simulink model "Copy_of_modele"  (R2025b)
settings: Solver=VariableStepAuto  StartTime=0.0  StopTime=100  RelTol=1e-3
values from neighbouring files (symbols this model uses):
  Axy = 0.0    (= 0)    [PropKtKq.m]    (also in variables_procom.m = prop.Axy)
  Cxy = 0.0    (= 0)    [PropKtKq.m]    (also in variables_procom.m = prop.Cxy)
  D = 0.0    (= 0)    [PropKtKq.m]    (also in variables_procom.m = prop.D)
  eta_mt = 0.4    [variables_procom.m]
  Jprop = Jmt/R^2    (= 19.35886398)    [variables_procom.m]
  m = 0.0    (= 0)    [Hulldyn.m]    (also in variables_procom.m = 250000)
  ma = 123434    [variables_procom.m]
  Pe = 5    [variables_procom.m]
  Py = 60    [variables_procom.m]
  R = 1/2.953    (= 0.338638672536)    [variables_procom.m]
  tau_mt = 0.4    [variables_procom.m]
  Tc = 0.0    (= 0)    [Hulldyn.m]    (also in variables_procom.m = 5800)
  th = 0.0    (= 0)    [Hulldyn.m]    (also in PropKtKq.m; variables_procom.m = hull.th)
  wh = 0.0    (= 0)    [Hulldyn.m]    (also in PropKtKq.m; variables_procom.m = hull.wh)
  x = 0.0    (= 0)    [PropKtKq.m]    (also in variables_procom.m = prop.x)
  y = 0.0    (= 0)    [PropKtKq.m]    (also in variables_procom.m = prop.y)
libraries: slpidlib x1
settings Model: Creator=leagr  LastModifiedBy=flo

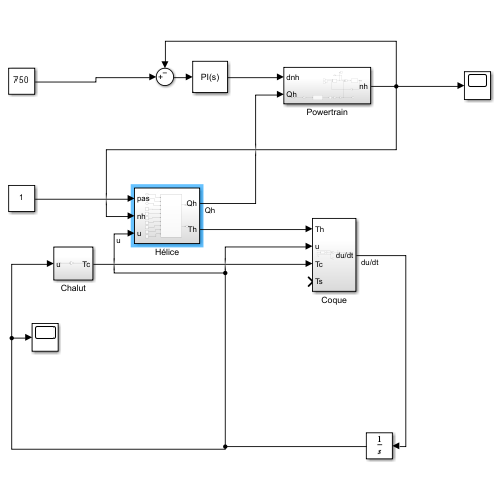
[thumbnail: Simulink's stored preview of the top-level diagram]
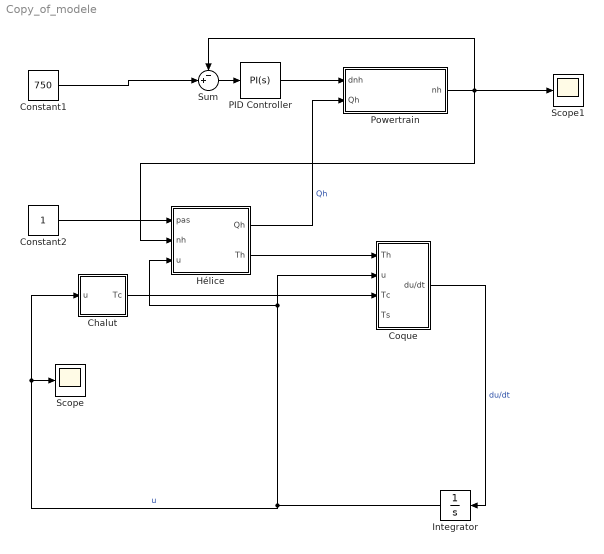
== system Copy_of_modele ==
  Chalut : Subsystem
  Constant1 : Constant  Value=750
  Constant2 : Constant
  Coque : Subsystem
  Hélice : Subsystem
  Integrator : Integrator
  PID Controller : slpidlib/PID Controller  Controller=PI  Form=Parallel  TimeDomain=Continuous-time  UseExternalTs=off  SampleTime=-1  IntegratorMethod=Forward Euler  FilterMethod=Forward Euler  ControllerParametersSource=internal  P=2.47620344962392  I=0.00577839793928918  UseKiTs=off  D=0  UseExternalDerivativeSource=off  N=100  UseFilter=on  TunerSelectOption=Transfer Function Based (PID Tuner App)  InitialConditionSource=internal  InitialConditionForIntegrator=0  InitialConditionForFilter=0  DifferentiatorICPrevScaledInput=0  ExternalReset=none  TrackingMode=off  Kt=1  LimitOutput=off  SatLimitsSource=internal  UpperSaturationLimit=inf  LowerSaturationLimit=-inf  LinearizeAsGain=on  AntiWindupMode=none  Kb=1  LimitIntegrator=off  UpperIntegratorSaturationLimit=inf  LowerIntegratorSaturationLimit=-inf  POutMin=[]  POutMax=[]  IOutMin=[]  IOutMax=[]  DOutMin=[]  DOutMax=[]  NOutMin=[]  NOutMax=[]  SumOutMin=[]  SumOutMax=[]  SaturationOutMin=[]  SaturationOutMax=[]  PParamMin=[]  PParamMax=[]  IParamMin=[]  IParamMax=[]  DParamMin=[]  DParamMax=[]  NParamMin=[]  NParamMax=[]  KbParamMin=[]  KbParamMax=[]  KtParamMin=[]  KtParamMax=[]  KbOutMin=[]  KbOutMax=[]  KtOutMin=[]  KtOutMax=[]  IntegratorOutMin=[]  IntegratorOutMax=[]  FilterOutMin=[]  FilterOutMax=[]  SumI1OutMin=[]  SumI1OutMax=[]  SumI2OutMin=[]  SumI2OutMax=[]  SumI3OutMin=[]  SumI3OutMax=[]  SumI4OutMin=[]  SumI4OutMax=[]  SumDOutMin=[]  SumDOutMax=[]  DifferentiatorOutMin=[]  DifferentiatorOutMax=[]  FilterDiffOutCoefMin=[]  FilterDiffOutCoefMax=[]  ReciprocalOutMin=[]  ReciprocalOutMax=[]  SumDenOutMin=[]  SumDenOutMax=[]  SumNumOutMin=[]  SumNumOutMax=[]  DivideOutMin=[]  DivideOutMax=[]  UdiffTsProdOutMin=[]  UdiffTsProdOutMax=[]  NTsProdOutMin=[]  NTsProdOutMax=[]  UintegralTsProdOutMin=[]  UintegralTsProdOutMax=[]  UngainTsProdOutMin=[]  UngainTsProdOutMax=[]  ClampingZeroOutDataTypeStr=Inherit: Inherit via back propagation  ClampingZeroOutMin=[]  ClampingZeroOutMax=[]  FilterDenConstantOutDataTypeStr=Inherit: Inherit via back propagation  FilterDenConstantOutMin=[]  FilterDenConstantOutMax=[]  PCopyOutDataTypeStr=Inherit: Inherit via back propagation  PCopyOutMin=[]  PCopyOutMax=[]  NCopyOutDataTypeStr=Inherit: Inherit via back propagation  NCopyOutMin=[]  NCopyOutMax=[]  IntegratorContinuousStateAttributes=''  IntegratorStateMustResolveToSignalObject=off  IntegratorRTWStateStorageClass=Auto  FilterContinuousStateAttributes=''  FilterStateMustResolveToSignalObject=off  FilterRTWStateStorageClass=Auto  ParallelPVariant=InternalParameters  IdealPVariant=Disabled  IVariant=InternalParameters  DVariant=Disabled  IntegratorVariant=Continuous  SatVariant=Disabled  AWVariant=Passthrough  PCopyVariant=Disabled  TRVariant=Disabled  FdbkBlocksVariant=Forward  IdealPFdbkVariant=Disabled  SatFdbkVariant=Disabled  DerivativeFilterVariant=Disabled  NVariant=Disabled  NCopyVariant=Disabled_SignalSpec  FilterICVariant=Disabled  IntegratorICVariant=InternalICs  ExternalResetVariant=Disabled  TRSumVariant=Passthrough  SumFdbkVariant=Disabled  SumVariant=Sum_PI  TsampFilterVariant=InternalTs  TsampNgainVariant=Passthrough  TsampIntegralVariant=Disabled_SignalSpec  ExternalSaturationOutDataTypeStr=Inherit: Same as second input  DerivativeSourceVariant=Disabled  PreIntVariant=InternalPreInt
  Powertrain : Subsystem
  Scope : Scope
      settings: ActiveDisplayYMinimum=-0.12811247147162838  ActiveDisplayYMaximum=1.1530122432446557
  Scope1 : Scope
      settings: ActiveDisplayYMinimum=-0.837262350749306  ActiveDisplayYMaximum=7.5353611567437557  DataLoggingVariableName=ScopeData3
  Sum : Sum  Inputs=-+|
  wires:
  Constant2/1 -> Hélice/1(pas)
  Constant1/1 -> Sum/2
  Sum/1 -> PID Controller/1
  PID Controller/1 -> Powertrain/1(dnh)
  Chalut/1(Tc) -> Coque/3(Tc)
  Powertrain/1(nh) -> Hélice/2(nh), Scope1/1, Sum/1
  Hélice/1(Qh) -> Powertrain/2(Qh)  "Qh"
  Hélice/2(Th) -> Coque/1(Th)
  Integrator/1 -> Chalut/1(u), Scope/1, Coque/2(u), Hélice/3(u)  "u"
  Coque/1(du/dt) -> Integrator/1  "du/dt"

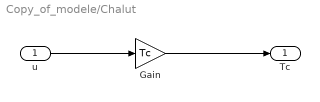
== system Copy_of_modele/Chalut ==
  u : Inport
  Gain : Gain  Gain=Tc
  Tc : Outport
  wires:
  u/1 -> Gain/1
  Gain/1 -> Tc/1

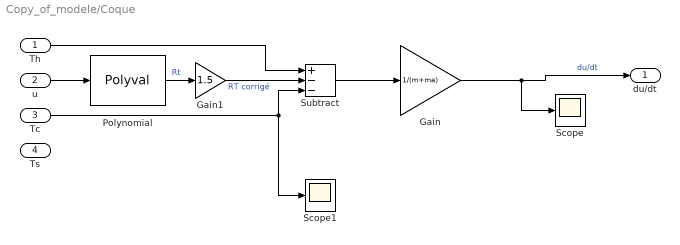
== system Copy_of_modele/Coque ==
  Th : Inport
  u : Inport  Port=2
  Tc : Inport  Port=3
  Ts : Inport  Port=4
  Gain : Gain  Gain=1/(m+ma)
  Gain1 : Gain  Gain=1.5
  Polynomial : Polyval  Coefs=[768.9,-3894,6949.8,-271.6]
  Scope : Scope
      settings: ActiveDisplayYMinimum=-1  ActiveDisplayYMaximum=1
  Scope1 : Scope
      settings: ActiveDisplayYMinimum=-1  ActiveDisplayYMaximum=1  DataLoggingVariableName=ScopeData2
  Subtract : Sum  Inputs=+--
  du/dt : Outport
  wires:
  Subtract/1 -> Gain/1
  Polynomial/1 -> Gain1/1  "Rt"
  Tc/1 -> Scope1/1, Subtract/3
  Gain/1 -> Scope/1, du/dt/1  "du/dt"
  Gain1/1 -> Subtract/2  "RT corrigé"
  u/1 -> Polynomial/1
  Th/1 -> Subtract/1

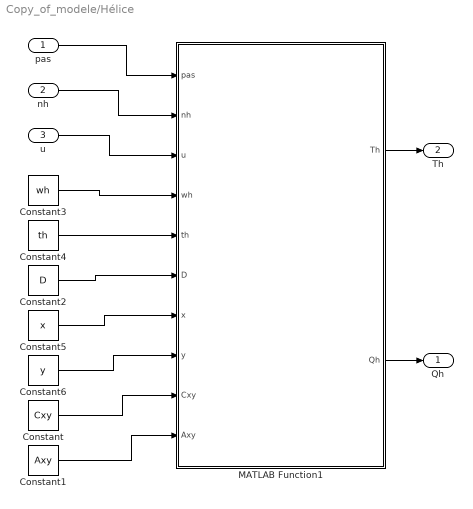
== system Copy_of_modele/Hélice ==
  pas : Inport
  nh : Inport  Port=2
  u : Inport  Port=3
  Constant : Constant  Value=Cxy
  Constant1 : Constant  Value=Axy
  Constant2 : Constant  Value=D
  Constant3 : Constant  Value=wh
  Constant4 : Constant  Value=th
  Constant5 : Constant  Value=x
  Constant6 : Constant  Value=y
  MATLAB Function1 : MATLAB Function  TreatAsAtomicUnit=on
  Qh : Outport
  Th : Outport  Port=2
  wires:
  pas/1 -> MATLAB Function1/1(pas)
  nh/1 -> MATLAB Function1/2(nh)
  Constant/1 -> MATLAB Function1/9(Cxy)
  u/1 -> MATLAB Function1/3(u)
  Constant3/1 -> MATLAB Function1/4(wh)
  Constant4/1 -> MATLAB Function1/5(th)
  Constant1/1 -> MATLAB Function1/10(Axy)
  Constant2/1 -> MATLAB Function1/6(D)
  Constant5/1 -> MATLAB Function1/7(x)
  Constant6/1 -> MATLAB Function1/8(y)
  MATLAB Function1/2(Qh) -> Qh/1
  MATLAB Function1/1(Th) -> Th/1

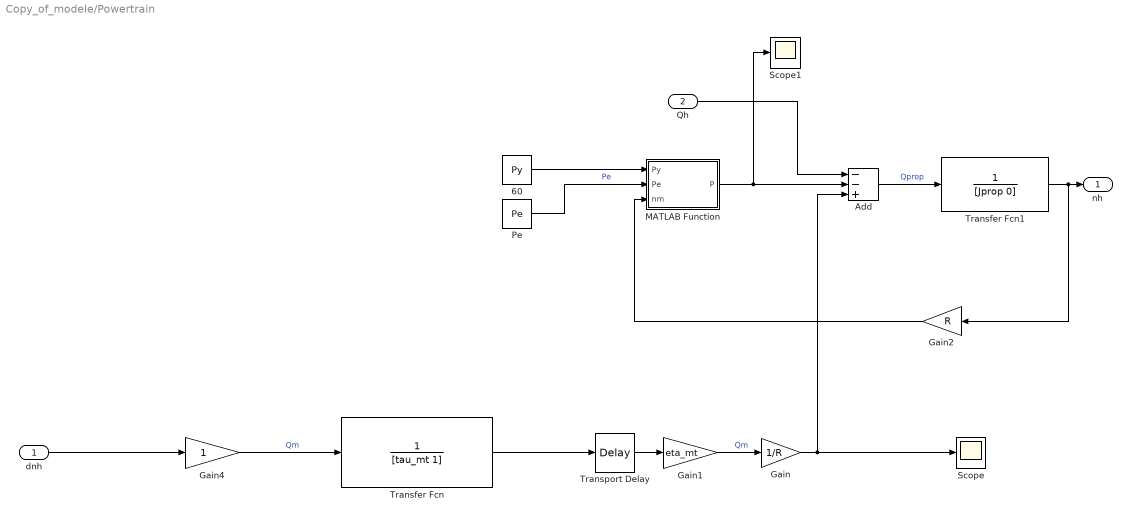
== system Copy_of_modele/Powertrain ==
  dnh : Inport
  Qh : Inport  Port=2
  60 : Constant  Value=Py
  Add : Sum  Inputs=--+
  Gain : Gain  Gain=1/R
  Gain1 : Gain  Gain=eta_mt
  Gain2 : Gain  Gain=R
  Gain4 : Gain
  MATLAB Function : MATLAB Function  TreatAsAtomicUnit=on
  Pe : Constant  Value=Pe
  Scope : Scope
      settings: ActiveDisplayYMinimum=-1  ActiveDisplayYMaximum=1
  Scope1 : Scope
      settings: ActiveDisplayYMinimum=-1  ActiveDisplayYMaximum=1  DataLoggingVariableName=ScopeData2
  Transfer Fcn : TransferFcn  Denominator=[tau_mt 1]
  Transfer Fcn1 : TransferFcn  Denominator=[Jprop 0]
  Transport Delay : TransportDelay
  nh : Outport
  wires:
  Qh/1 -> Add/1
  Add/1 -> Transfer Fcn1/1  "Qprop"
  Transfer Fcn1/1 -> Gain2/1, nh/1
  Transport Delay/1 -> Gain1/1
  Gain/1 -> Scope/1, Add/3
  Gain1/1 -> Gain/1  "Qm"
  Transfer Fcn/1 -> Transport Delay/1
  Gain4/1 -> Transfer Fcn/1  "Qm"
  dnh/1 -> Gain4/1
  Gain2/1 -> MATLAB Function/3(nm)
  60/1 -> MATLAB Function/1(Py)
  Pe/1 -> MATLAB Function/2(Pe)  "Pe"
  MATLAB Function/1(P) -> Scope1/1, Add/2

== matlab function Copy_of_modele/Hélice/MATLAB Function1 ==
  data: pas input; nh input; u input; Th output; Qh output; wh input; th input; D input; x input; y input; Cxy input; Axy input
function [Th,Qh]= fcn(pas, nh, u, wh, th ,D, x, y, Cxy, Axy)

    rho = 1025; % Masse volumique de l'eau
    
    % Conversion rad/s en tr/s pour les calculs
    Nh = nh/(2*pi);
    
    % Coefficient d'avance et rapport P/D
    J = u*(1-wh)/(D*Nh);
    P_D = pas/D;
    
    % Calcul des coefficients Kt et Kq pour ce point de fonctionnement
    Kt = 0.5; % dot(Axy, P_D.^x .* J.^y);
    Kq = 0.06; % dot(Cxy, P_D.^x .* J.^y);
    
    % Calcul de la poussée
    Th = (1-th)*Kt*rho*D^4*Nh^2;
    Qh = Kq*rho*D^5*Nh^2;

end

== matlab function Copy_of_modele/Powertrain/MATLAB Function ==
  data: Py input; P output; Pe input; nm input
function P = fcn(Py, Pe, nm)
threshold = 100; % On ne branche l'aternateur et les pompes qu'une fois
                 % un certain régime atteint.
eta_p = 0.5;
    if nm < threshold
        P = 0;
    else
        P = (Pe*eta_p+Py)/nm;
    end
